simulink model "Speed_Controller_Test"  (Simulink 7.2)
settings: Solver=ode4  SolverMode=SingleTasking  StartTime=0.0  StopTime=252  FixedStep=0.01  RelTol=1e-3
InitFcn:
  | tempomat_para
StopFcn:
  | clear;
values from neighbouring files (symbols this model uses):
  A = 1.9    [tempomat_para.m]
  a_Fzg_max = 2    [tempomat_para.m]
  a_Fzg_min = -2    [tempomat_para.m]
  cw = 0.32    [tempomat_para.m]
  gang = [1 2 3 4]    [tempomat_para.m]
  gang_vec = [1 2 3 4]    [tempomat_para.m]
  i_anteil = 5    [tempomat_para.m]
  i_d = 3.42    [tempomat_para.m]
  i_g = [3.91 2.17 1.37 1.00]    [tempomat_para.m]
  lambda_gang = [1.3 1.25  1.17  1.05]    [tempomat_para.m]
  m_Fzg = 1400    [tempomat_para.m]
  M_mot_max = [130 149 163 170 168 166 162 158 150 139 123 80]    [tempomat_para.m]
  M_mot_min = [0 -40]    [tempomat_para.m]
  n_mot0 = 1000    [tempomat_para.m]
  n_mot_max = 1000:500:6500    [tempomat_para.m]
  n_mot_min = [1000 6500]    [tempomat_para.m]
  p_anteil = 100    [tempomat_para.m]
  r_dyn = 0.28    [tempomat_para.m]
  rho = 1.202    [tempomat_para.m]
  t_sch = 0.2    [tempomat_para.m]
  TI = [block '/TI']    [PSTI_callback.m]
  v_Fzg_ms0 = 0    [tempomat_para.m]
undefined symbols (not defined in the file or in its folder): Drossel_mat, getdatatypespecs
libraries: simulink x116, fzgbib x3
(part 2 of 10)

== system Speed_Controller_Test/Validation and  Test Evaluation/R2 Speed Control velocity restoration time after simple  acceleration/deceleration/CC active + no target & Speed Control active & step of V_Des = |1|  with time periods >= 7s ==
  InOut Bus : Inport  OutDataType=sfix(16)  OutScaling=2^0
  Active : Constant  Value=2  OutDataType=sfix(16)  OutScaling=2^0
  Active + no target : Constant  Value=2  OutDataType=sfix(16)  OutScaling=2^0
  Bus Selector : BusSelector  OutputSignals=Inputs.v_Des,Inputs.CCMode,Inputs.Selection
  CC active & no target : Subsystem  mask(Range - Gap Absolute Tolerance){GorR=Range, AbsoluteTolerance=0}
      mask prompts: GorR "Use range or gap"; AbsoluteTolerance "Absolute Tolerance"
      mask help: Check that a signal stays inside a range or outside a gap around a reference signal. Specify the range or the gap absolute to the reference signal.
      mask init:
      | if max(get_param(gcb,'GorR') == ' ') % Gap
      |     helpVariable1 = '~=';
      | else % Range
      |     helpVariable1 = '==';
      | end
      | set_param([gcb '/Relational Operator'],'Operator',helpVariable1);
      mask StyleString: popup(Range|Gap  ),edit
      mask Display:
      | port_label('output',1,'A');
      | port_label('input',1,'Sig');
      | port_label('input',2,'Ref');
      | text(0.40,0.53,'+');
      | text(0.415,0.46,'-');
      | text(0.5,0.5,num2str(AbsoluteTolerance));
      | text(0.05,0.5,helpVariable1);
  CC active & no target1 : Subsystem  mask(Range - Gap Absolute Tolerance){GorR=Range, AbsoluteTolerance=0}
      mask prompts: GorR "Use range or gap"; AbsoluteTolerance "Absolute Tolerance"
      mask help: Check that a signal stays inside a range or outside a gap around a reference signal. Specify the range or the gap absolute to the reference signal.
      mask init:
      | if max(get_param(gcb,'GorR') == ' ') % Gap
      |     helpVariable1 = '~=';
      | else % Range
      |     helpVariable1 = '==';
      | end
      | set_param([gcb '/Relational Operator'],'Operator',helpVariable1);
      mask StyleString: popup(Range|Gap  ),edit
      mask Display:
      | port_label('output',1,'A');
      | port_label('input',1,'Sig');
      | port_label('input',2,'Ref');
      | text(0.40,0.53,'+');
      | text(0.415,0.46,'-');
      | text(0.5,0.5,num2str(AbsoluteTolerance));
      | text(0.05,0.5,helpVariable1);
  PS : Subsystem  mask(Feature layer: preconditions synchronization){NoTI=3, NoTDD=0, NoTID=0, TIdel=[0  0  0], TDDdel=[]}
      mask prompts: NoTI "Time-independent features identifiable with or without a delay (TI)"; NoTDD "Triggered features identifiable with determinate delay or without a delay (TDD)"; NoTID "Triggered features identifiable with indeterminate delay (TID)"; TIdel "Time-independent features delays (in time steps). E.g. [0 1 0] for 3 features"; TDDdel "Triggered features delays (in time steps). E.g. [0 0] for 2 features"
      mask help: Use this block for synchronizing the precondition features. For changing the block inputs, use the parameters below. The output must be used for assertions activation.
      mask init:
      | PS_init(gcb);
      mask StyleString: popup(0|1|2|3|4|5|6|7|8|9),popup(0|1|2|3|4|5|6|7|8|9),popup(0|1|2|3|4|5|6|7|8|9),edit,edit
      mask CallbackString:
      | PSTI_callback(gcb);|PSTDD_callback(gcb);|PSTID_callback(gcb);|NoTI = str2double(get_param(gcb,'NoTI'));
      | TIdel = str2num(get_param(gcb,'TIdel'));
      | if NoTI ~= length(TIdel) && NoTI ~= 0
      |     error(['The number of delays entered (' num2str(length(TIdel)) ') does not correspond to the above specified number of time-independent features (' num2str(NoTI) ').']);
      | end|NoTDD = str2double(get_param(gcb,'NoTDD'));
      | TDDdel = str2num(get_param(gcb,'TDDdel'));
      | if NoTDD ~= length(TDDdel) && NoTDD ~= 0
      |     error(['The number of delays entered (' num2str(length(TDDdel)) ') does not correspond to the above specified number of triggered features with constant delay (' num2str(NoTDD) ').']);
      | end
  Scope1 : Scope  NumInputPorts=3
      settings: TimeRange=120  YMin=-0.003370786516853574~-5~-5  YMax=0.3966292134831465~5~5  SaveName=ScopeData5  MaxDataPoints=5000000
  Speed Control active : Subsystem  mask(Range - Gap Absolute Tolerance){GorR=Range, AbsoluteTolerance=0}
      mask prompts: GorR "Use range or gap"; AbsoluteTolerance "Absolute Tolerance"
      mask help: Check that a signal stays inside a range or outside a gap around a reference signal. Specify the range or the gap absolute to the reference signal.
      mask init:
      | if max(get_param(gcb,'GorR') == ' ') % Gap
      |     helpVariable1 = '~=';
      | else % Range
      |     helpVariable1 = '==';
      | end
      | set_param([gcb '/Relational Operator'],'Operator',helpVariable1);
      mask StyleString: popup(Range|Gap  ),edit
      mask Display:
      | port_label('output',1,'A');
      | port_label('input',1,'Sig');
      | port_label('input',2,'Ref');
      | text(0.40,0.53,'+');
      | text(0.415,0.46,'-');
      | text(0.5,0.5,num2str(AbsoluteTolerance));
      | text(0.05,0.5,helpVariable1);
  Step with step size=|1|  and time periods >= 6s detection : Subsystem  mask(Complete step detection){Param=0}
      mask prompts: Param "Mask Parameter 1:"
  true : Constant  OutDataType=sfix(16)  OutScaling=2^0
  Activate : Outport  OutDataType=sfix(16)  OutScaling=2^0
  wires:
  PS/1(Precond) -> Activate/1
  InOut Bus/1 -> Bus Selector/1
  Bus Selector/1 -> Step with step size=|1|  and time periods >= 6s detection/1(Step)  "<v_Des>"
  Bus Selector/2 -> CC active & no target/1(Signal)  "<CCMode>"
  Active + no target/1 -> CC active & no target/2(Reference)
  Active/1 -> Speed Control active/2(Reference)
  Bus Selector/3 -> Speed Control active/1(Signal)  "<Selection>"
  Step with step size=|1|  and time periods >= 6s detection/1(Complete step) -> CC active & no target1/1(Signal)
  true/1 -> CC active & no target1/2(Reference)
  CC active & no target1/1(Activate) -> PS/1(A TI1)
  CC active & no target/1(Activate) -> PS/2(A TI2)
  Speed Control active/1(Activate) -> PS/3(A TI3)

== system Speed_Controller_Test/Validation and  Test Evaluation/R2 Speed Control velocity restoration time after simple  acceleration/deceleration/after (6 seconds)  |V_Des-V_Vhcl <= 1.4| ==
  Precond : Inport  OutDataType=sfix(16)  OutScaling=2^0
  InOut Bus : Inport  Port=2  OutDataType=sfix(16)  OutScaling=2^0
  " " : Subsystem  mask(Bound){cm=<=, Lower=1, Upper=0, Ass=[1 2], Pre=[1 2], Req=[1 2]}
      mask prompts: cm "Comparison method:"; Upper "Mask Parameter 3:"; Req "Mask Parameter 6:"
      mask help:
      | Compare a signal with a reference using the specified comparison method.
      |
      | Output verdict V and lower (LL) and upper (UL) limits for reporting.
      |
      | For '==' or '~=' use "Range - Gap"
      mask init: same as Speed_Controller_Test/Validation and  Test Evaluation/R1 Speed Control step response/Maximum overshoot < 5 &  Steady state error < 5/Maximum overshoot < 5
      mask StyleString: popup(>|>=|<=|<),edit,edit,edit,edit,edit
      mask Display:
      | port_label('output', 1, ['V']);
      | port_label('input', 1, 'Sig');
      | port_label('input', 2, 'Ref');
      | text(0.05,0.5,get_param(get_param([get_param(gcb,'Parent') '/' get_param(gcb,'Name') '/Relational Operator'],'handle'),'Operator'));
  Bus Creator : BusCreator  Inputs=1
  Bus Selector : BusSelector  OutputSignals=Inputs.v_Des,Outputs.v_Vhcl
  Bus Selector{1..4} (4 alike) : BusSelector  OutputSignals=Local verdict
  PAS1 : Subsystem  mask{AFT=TI, AFD=600}
      mask prompts: AFT "Assertion feature type:"; AFD "Assertion feature delay (in time steps)"
      mask init:
      | PAS_init(gcb);
      mask StyleString: popup(TI|TDD|TID),edit
      mask CallbackString: PAS_callback(gcb);|
  PAS2 : Subsystem  mask{AFT=TI, AFD=600}
      mask prompts: AFT "Assertion feature type:"; AFD "Assertion feature delay (in time steps)"
      mask init:
      | PAS_init(gcb);
      mask StyleString: popup(TI|TDD|TID),edit
      mask CallbackString: PAS_callback(gcb);|
  R = 2 : Subsystem
  Scope : Scope  NumInputPorts=5
      settings: YMin=-5~-5~-5~80~0  YMax=5~5~5~107.5~110  SaveName=ScopeData2  MaxDataPoints=5000000
  t1 : Constant  Value=1.4  OutDataType=sfix(16)  OutScaling=2^0
  t2 : Constant  OutDataType=sfix(16)  OutScaling=2^0
  within(20 sec)1 : Subsystem  mask(Bound){cm=<=, Lower=1, Upper=0, Ass=[1 2], Pre=[1 2], Req=[1 2]}
      mask prompts: cm "Comparison method:"; Upper "Mask Parameter 3:"; Req "Mask Parameter 6:"
      mask help:
      | Compare a signal with a reference using the specified comparison method.
      |
      | Output verdict V and lower (LL) and upper (UL) limits for reporting.
      |
      | For '==' or '~=' use "Range - Gap"
      mask init: same as Speed_Controller_Test/Validation and  Test Evaluation/R1 Speed Control step response/Maximum overshoot < 5 &  Steady state error < 5/Maximum overshoot < 5
      mask StyleString: popup(>|>=|<=|<),edit,edit,edit,edit,edit
      mask Display:
      | port_label('output', 1, ['V']);
      | port_label('input', 1, 'Sig');
      | port_label('input', 2, 'Ref');
      | text(0.05,0.5,get_param(get_param([get_param(gcb,'Parent') '/' get_param(gcb,'Name') '/Relational Operator'],'handle'),'Operator'));
  |V_Des-V_Vhcl| : Subsystem
  VF info : Outport  OutDataType=sfix(16)  OutScaling=2^0
  wires:
  t1/1 -> " "/2(Reference)
  " "/1(V) -> Bus Selector1/1, PAS1/2(V)
  InOut Bus/1 -> |V_Des-V_Vhcl|/1(InOut Bus), Bus Selector/1, R = 2/2(In2)
  Bus Creator/1 -> VF info/1
  Precond/1 -> PAS1/1(Precond), PAS2/1(Precond), R = 2/1(In1)
  PAS1/1(VF Info) -> Bus Creator/1, Bus Selector2/1
  |V_Des-V_Vhcl|/1(Out1) -> " "/1(Signal)
  t2/1 -> within(20 sec)1/2(Reference)
  within(20 sec)1/1(V) -> Bus Selector4/1, PAS2/2(V)
  R = 2/1(Out1) -> within(20 sec)1/1(Signal), Scope/3
  Bus Selector4/1 -> Scope/1  "<Local verdict>"
  PAS2/1(VF Info) -> Bus Selector3/1
  Bus Selector3/1 -> Scope/2  "<Local verdict>"

== system Speed_Controller_Test/Speed control/Compute SUC inputs/neg_Beschleunigungsbegrenzung/Reset M_Br2 ==
  M_Br_n : Inport  OutDataType=sfix(16)  OutScaling=2^0
  a_Fzg_mss : Inport  Port=2  OutDataType=sfix(16)  OutScaling=2^0
  Enable : EnablePort
  Constant1 : Constant  Value=a_Fzg_min  OutDataType=sfix(16)  OutScaling=2^0
  Constant2 : Constant  Value=10  OutDataType=sfix(16)  OutScaling=2^0
  Data Store Write : DataStoreWrite  DataStoreName=M_Br2  SampleTime=-1
  Product : Product  OutDataType=sfix(16)  OutScaling=2^0  SaturateOnIntegerOverflow=on  InputSameDT=on  OutDataTypeStr=Inherit: Same as first input
  Sum : Sum  OutDataType=sfix(16)  OutScaling=2^0  SaturateOnIntegerOverflow=on  InputSameDT=on  OutDataTypeStr=Inherit: Same as first input
  Sum1 : Sum  Inputs=+-  OutDataType=sfix(16)  OutScaling=2^0  SaturateOnIntegerOverflow=on  InputSameDT=on  OutDataTypeStr=Inherit: Same as first input
  wires:
  Sum/1 -> Data Store Write/1
  M_Br_n/1 -> Sum/1
  Sum1/1 -> Product/2
  a_Fzg_mss/1 -> Sum1/1
  Constant1/1 -> Sum1/2
  Constant2/1 -> Product/1
  Product/1 -> Sum/2

== system Speed_Controller_Test/Speed control/Compute SUC inputs/pos_Beschleunigungsbegrenzung/Reset M_Mot2 ==
  M_Mot_n : Inport  OutDataType=sfix(16)  OutScaling=2^0
  Enable : EnablePort
  Data Store Write : DataStoreWrite  DataStoreName=M_Mot2  SampleTime=-1
  wires:
  M_Mot_n/1 -> Data Store Write/1

== system Speed_Controller_Test/Speed control/Speed controller/Stoergroessenkompensation/Luft- und Rollwiderstand ==
  note: Keine Steigung beruecksichtigt
  v_Fzg : Inport  OutDataType=sfix(16)  OutScaling=2^0
  F_L Berechnung : Fcn  Expr=u*rho*A/2*cw
  F_R Berechnung : Fcn  Expr=(u>0.1)*f_r*m_Fzg*g
  Fcn : Fcn  Expr=u*r_dyn
  Product : Product  OutDataType=sfix(16)  OutScaling=2^0  SaturateOnIntegerOverflow=on  InputSameDT=on  OutDataTypeStr=Inherit: Same as first input
  Sum : Sum  OutDataType=sfix(16)  OutScaling=2^0  SaturateOnIntegerOverflow=on  InputSameDT=on  OutDataTypeStr=Inherit: Same as first input
  M_G : Outport  OutDataType=sfix(16)  OutScaling=2^0  InitialOutput=0
  wires:
  Product/1 -> F_L Berechnung/1
  v_Fzg/1 -> Product/2, Product/1, F_R Berechnung/1
  F_R Berechnung/1 -> Sum/2
  F_L Berechnung/1 -> Sum/1
  Sum/1 -> Fcn/1
  Fcn/1 -> M_G/1

== system Speed_Controller_Test/Speed control/Speed controller/Stoergroessenkompensation/Sollverhalten Fahrzeug mit P-Regler1 ==
  v_soll : Inport  OutDataType=sfix(16)  OutScaling=2^0
  v_Fzg : Inport  Port=2  OutDataType=sfix(16)  OutScaling=2^0
  GR_aktiv_l : Inport  Port=3  OutDataType=sfix(16)  OutScaling=2^0
  1/T : Fcn  Expr=1/u
  Grenze3 : Constant  Value=r_dyn*m_Fzg/p_anteil  OutDataType=sfix(16)  OutScaling=2^0
  Grenze4 : Constant  Value=0.1  OutDataType=sfix(16)  OutScaling=2^0
  Integrator : Integrator  InitialCondition=v_Fzg_ms0
  Product : Product  OutDataType=sfix(16)  OutScaling=2^0  SaturateOnIntegerOverflow=on  InputSameDT=on  OutDataTypeStr=Inherit: Same as first input
  Reglerabweichung : Sum  Inputs=-+  OutDataType=sfix(16)  OutScaling=2^0  SaturateOnIntegerOverflow=on  InputSameDT=on  OutDataTypeStr=Inherit: Same as first input
  Switch : Switch  Threshold=0.5  SaturateOnIntegerOverflow=on  InputSameDT=on
  Switch1 : Switch  Threshold=0.5  SaturateOnIntegerOverflow=on  InputSameDT=on
  v_Fzg1 : Outport  OutDataType=sfix(16)  OutScaling=2^0  InitialOutput=0
  wires:
  GR_aktiv_l/1 -> Switch1/2, Switch/2
  v_Fzg/1 -> Switch1/3
  v_soll/1 -> Switch1/1
  Switch1/1 -> Reglerabweichung/2
  Grenze3/1 -> Switch/1
  Grenze4/1 -> Switch/3
  1/T/1 -> Product/2
  Reglerabweichung/1 -> Product/1
  Switch/1 -> 1/T/1
  Product/1 -> Integrator/1
  Integrator/1 -> Reglerabweichung/1, v_Fzg1/1

== system Speed_Controller_Test/Speed control/Vehicle model/Fahrzeugmodell/Drosselklappenstellung ==
  n_mot : Inport  OutDataType=sfix(16)  OutScaling=2^0
  M_Mot_b : Inport  Port=2  OutDataType=sfix(16)  OutScaling=2^0
  schalt_l : Inport  Port=3  OutDataType=sfix(16)  OutScaling=2^0
  Constant : Constant  Value=0  OutDataType=sfix(16)  OutScaling=2^0
  Constant1 : Constant  Value=n_mot0+100  OutDataType=sfix(16)  OutScaling=2^0
  Constant2 : Constant  Value=0  OutDataType=sfix(16)  OutScaling=2^0
  Drosselklappenkennfeld : Lookup2D  RowIndex=n_Mot_vec  ColumnIndex=M_Mot_vec  Table=Drossel_mat  OutDataType=sfix(16)  OutScaling=2^0  SaturateOnIntegerOverflow=on  InputSameDT=on
  Logical Operator : Logic
  Logical Operator1 : Logic  Operator=OR
  PT1 Filterung : TransferFcn  Denominator=[0.1 1]
  Relational Operator : RelationalOperator  InputSameDT=on
  Relational Operator1 : RelationalOperator  Operator=<=  InputSameDT=on
  Saturation : Saturate  UpperLimit=90  LowerLimit=0
  Switch : Switch  Threshold=0.5  SaturateOnIntegerOverflow=on  InputSameDT=on
  damit bei Vollast 90 Grad : Fcn  Expr=u+3
  DK_Stellung [Grad] : Outport  OutDataType=sfix(16)  OutScaling=2^0  InitialOutput=0
  wires:
  Relational Operator1/1 -> Logical Operator/2
  Relational Operator/1 -> Logical Operator/1
  Logical Operator/1 -> Logical Operator1/1
  schalt_l/1 -> Logical Operator1/2
  Constant/1 -> Switch/1
  Logical Operator1/1 -> Switch/2
  Constant2/1 -> Relational Operator1/2
  Constant1/1 -> Relational Operator/2
  Saturation/1 -> PT1 Filterung/1
  PT1 Filterung/1 -> DK_Stellung [Grad]/1
  Switch/1 -> Saturation/1
  M_Mot_b/1 -> Relational Operator1/1, Drosselklappenkennfeld/2
  n_mot/1 -> Relational Operator/1, Drosselklappenkennfeld/1
  Drosselklappenkennfeld/1 -> damit bei Vollast 90 Grad/1
  damit bei Vollast 90 Grad/1 -> Switch/3

== system Speed_Controller_Test/Speed control/Vehicle model/Fahrzeugmodell/Fahrwiderstaende ==
  note: Widerstandskraefte
  note: Keine Steigung beruecksichtigt
  M_Mot_b : Inport  OutDataType=sfix(16)  OutScaling=2^0
  M_Br_b : Inport  Port=2  OutDataType=sfix(16)  OutScaling=2^0
  Gang_w : Inport  Port=3  OutDataType=sfix(16)  OutScaling=2^0
  v_Fzg_ms : Inport  Port=4  OutDataType=sfix(16)  OutScaling=2^0
  F_A Berechnung ausgekuppelt : Constant  Value=0  OutDataType=sfix(16)  OutScaling=2^0
  F_A Berechnung eingekuppelt : Fcn  Expr=u[1]*u[2]*i_d/r_dyn
  F_Brems Berechnung : Fcn  Expr=(u[1]>0)*u[2]/r_dyn
  F_L Berechnung : Fcn  Expr=u*rho*A/2*cw
  F_R Berechnung : Fcn  Expr=(u>0.1)*f_r*m_Fzg*g
  Gesamtgetriebe- uebersetzung : Fcn  Expr=u*i_d
  Getriebeuebersetzung : Lookup  InputValues=gang  Table=i_g  OutDataType=sfix(16)  OutScaling=2^0  SaturateOnIntegerOverflow=on
  Mux : Mux  Inputs=2
  Mux1 : Mux  Inputs=2
  Product : Product  OutDataType=sfix(16)  OutScaling=2^0  SaturateOnIntegerOverflow=on  InputSameDT=on  OutDataTypeStr=Inherit: Same as first input
  Schaltdauer : Subsystem
  Switch : Switch  Threshold=0.5  SaturateOnIntegerOverflow=on  InputSameDT=on
  Zeit bis Gang  eingelegt ist : TransportDelay  DelayTime=t_sch  InitialOutput=1
  tw3 : ToWorkspace  VariableName=k_l  SaveFormat=Array
      settings: MaxDataPoints=speicher
  F_A : Outport  OutDataType=sfix(16)  OutScaling=2^0  InitialOutput=0
  F_L : Outport  Port=2  OutDataType=sfix(16)  OutScaling=2^0  InitialOutput=0
  F_R : Outport  Port=3  OutDataType=sfix(16)  OutScaling=2^0  InitialOutput=0
  F_Brems : Outport  Port=4  OutDataType=sfix(16)  OutScaling=2^0  InitialOutput=0
  i_gesamt : Outport  Port=5  OutDataType=sfix(16)  OutScaling=2^0  InitialOutput=0
  Gang_i : Outport  Port=6  OutDataType=sfix(16)  OutScaling=2^0  InitialOutput=0
  schalt_l : Outport  Port=7  OutDataType=sfix(16)  OutScaling=2^0  InitialOutput=0
  wires:
  F_L Berechnung/1 -> F_L/1
  Product/1 -> F_L Berechnung/1
  v_Fzg_ms/1 -> Product/2, Product/1, F_R Berechnung/1, Mux1/1
  F_Brems Berechnung/1 -> F_Brems/1
  F_R Berechnung/1 -> F_R/1
  Mux1/1 -> F_Brems Berechnung/1
  M_Br_b/1 -> Mux1/2
  Schaltdauer/1(k_l) -> schalt_l/1, Switch/2, tw3/1
  F_A Berechnung eingekuppelt/1 -> Switch/3
  M_Mot_b/1 -> Mux/2
  Mux/1 -> F_A Berechnung eingekuppelt/1
  Gesamtgetriebe- uebersetzung/1 -> i_gesamt/1
  Getriebeuebersetzung/1 -> Mux/1, Gesamtgetriebe- uebersetzung/1
  Switch/1 -> F_A/1
  Gang_w/1 -> Getriebeuebersetzung/1, Schaltdauer/1(Gang_w), Zeit bis Gang  eingelegt ist/1
  F_A Berechnung ausgekuppelt/1 -> Switch/1
  Zeit bis Gang  eingelegt ist/1 -> Gang_i/1

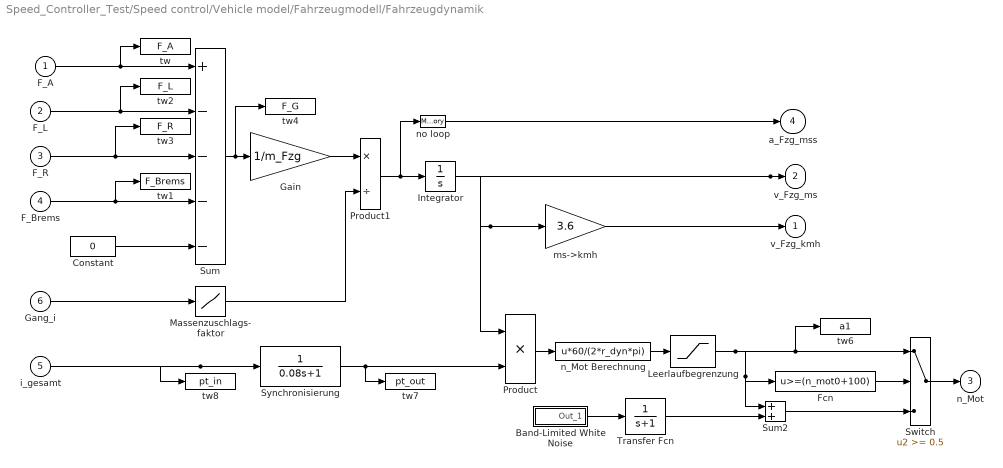
== system Speed_Controller_Test/Speed control/Vehicle model/Fahrzeugmodell/Fahrzeugdynamik ==
  F_A : Inport  OutDataType=sfix(16)  OutScaling=2^0
  F_L : Inport  Port=2  OutDataType=sfix(16)  OutScaling=2^0
  F_R : Inport  Port=3  OutDataType=sfix(16)  OutScaling=2^0
  F_Brems : Inport  Port=4  OutDataType=sfix(16)  OutScaling=2^0
  i_gesamt : Inport  Port=5  OutDataType=sfix(16)  OutScaling=2^0
  Gang_i : Inport  Port=6  OutDataType=sfix(16)  OutScaling=2^0
  Band-Limited White Noise : Subsystem  mask(Continuous White Noise.){@1=[3], @2=0.2, @3=[23341]}
      mask prompts: @1 "Noise Power:"; @2 "Sample Time:"; @3 "Seed"
      mask help:
      | White noise for continuous (s-domain) systems.
      | Band-limited using zero-order-hold.
      mask init:
      | Cov = @1; Ts = @2; seed = @3; r = rand(1,12); r2 = [r(1),r;r,r(12)]; t =[1:13;1:13];
      mask Help: Implemented using white noise into Zero-Order Hold block. The seed and power can be vectors of the same length to produce a vector of white noise sources. For faster simulation, set sample time to the highest value possible but in accordance with the fastest dynamics of system.
      mask Display: plot(t(:),r2(:))
  Constant : Constant  Value=0  OutDataType=sfix(16)  OutScaling=2^0
  Fcn : Fcn  Expr=u>=(n_mot0+100)
  Gain : Gain  Gain=1/m_Fzg  ParameterDataType=sfix(16)  ParameterScaling=2^0  OutDataType=sfix(16)  OutScaling=2^0  SaturateOnIntegerOverflow=on  OutDataTypeStr=Inherit: Same as input  ParamDataTypeStr=Inherit: Same as input
  Integrator : Integrator  InitialCondition=v_Fzg_ms0  UpperSaturationLimit=100  LowerSaturationLimit=0
  Leerlaufbegrenzung : Saturate  UpperLimit=7000  LowerLimit=n_mot0
  Massenzuschlags- faktor : Lookup  InputValues=gang_vec  Table=lambda_gang  OutDataType=sfix(16)  OutScaling=2^0  SaturateOnIntegerOverflow=on
  Product : Product  OutDataType=sfix(16)  OutScaling=2^0  SaturateOnIntegerOverflow=on  InputSameDT=on  OutDataTypeStr=Inherit: Same as first input
  Product1 : Product  Inputs=*/  OutDataType=sfix(16)  OutScaling=2^0  SaturateOnIntegerOverflow=on  InputSameDT=on  OutDataTypeStr=Inherit: Same as first input
  Sum : Sum  Inputs=+----  OutDataType=sfix(16)  OutScaling=2^0  SaturateOnIntegerOverflow=on  InputSameDT=on  OutDataTypeStr=Inherit: Same as first input
  Sum2 : Sum  OutDataType=sfix(16)  OutScaling=2^0  SaturateOnIntegerOverflow=on  InputSameDT=on  OutDataTypeStr=Inherit: Same as first input
  Switch : Switch  Threshold=0.5  SaturateOnIntegerOverflow=on  InputSameDT=on
  Synchronisierung : TransferFcn  Denominator=[0.08 1]
  Transfer Fcn : TransferFcn  Denominator=[1 1]
  ms->kmh : Gain  Gain=3.6  ParameterDataType=sfix(16)  ParameterScaling=2^0  OutDataType=sfix(16)  OutScaling=2^0  SaturateOnIntegerOverflow=on  OutDataTypeStr=Inherit: Same as input  ParamDataTypeStr=Inherit: Same as input
  n_Mot Berechnung : Fcn  Expr=u*60/(2*r_dyn*pi)
  no loop : Memory
  tw : ToWorkspace  VariableName=F_A  SaveFormat=Array
      settings: MaxDataPoints=speicher
  tw1 : ToWorkspace  VariableName=F_Brems  SaveFormat=Array
      settings: MaxDataPoints=speicher
  tw2 : ToWorkspace  VariableName=F_L  SaveFormat=Array
      settings: MaxDataPoints=speicher
  tw3 : ToWorkspace  VariableName=F_R  SaveFormat=Array
      settings: MaxDataPoints=speicher
  tw4 : ToWorkspace  VariableName=F_G  SaveFormat=Array
      settings: MaxDataPoints=speicher
  tw6 : ToWorkspace  VariableName=a1  SaveFormat=Array
      settings: MaxDataPoints=speicher
  tw7 : ToWorkspace  VariableName=pt_out  SaveFormat=Array
      settings: MaxDataPoints=speicher
  tw8 : ToWorkspace  VariableName=pt_in  SaveFormat=Array
      settings: MaxDataPoints=speicher
  v_Fzg_kmh : Outport  OutDataType=sfix(16)  OutScaling=2^0  InitialOutput=0
  v_Fzg_ms : Outport  Port=2  OutDataType=sfix(16)  OutScaling=2^0  InitialOutput=0
  n_Mot : Outport  Port=3  OutDataType=sfix(16)  OutScaling=2^0  InitialOutput=0
  a_Fzg_mss : Outport  Port=4  OutDataType=sfix(16)  OutScaling=2^0  InitialOutput=0
  wires:
  Constant/1 -> Sum/5
  F_Brems/1 -> tw1/1, Sum/4
  F_R/1 -> Sum/3, tw3/1
  F_L/1 -> Sum/2, tw2/1
  F_A/1 -> tw/1, Sum/1
  ms->kmh/1 -> v_Fzg_kmh/1
  Integrator/1 -> Product/1, ms->kmh/1, v_Fzg_ms/1
  no loop/1 -> a_Fzg_mss/1
  Product/1 -> n_Mot Berechnung/1
  n_Mot Berechnung/1 -> Leerlaufbegrenzung/1
  Gang_i/1 -> Massenzuschlags- faktor/1
  Massenzuschlags- faktor/1 -> Product1/2
  Product1/1 -> no loop/1, Integrator/1
  Gain/1 -> Product1/1
  Sum/1 -> Gain/1, tw4/1
  Synchronisierung/1 -> Product/2, tw7/1
  i_gesamt/1 -> Synchronisierung/1, tw8/1
  Fcn/1 -> Switch/2
  Sum2/1 -> Switch/3
  Leerlaufbegrenzung/1 -> tw6/1, Switch/1, Sum2/1, Fcn/1
  Transfer Fcn/1 -> Sum2/2
  Band-Limited White Noise/1(Out_1) -> Transfer Fcn/1
  Switch/1 -> n_Mot/1

== system Speed_Controller_Test/TestData 1/R1 Speed Control step response/Complete step & CC active + no target & Speed Control active/Generate complete step ==
  Out Bus : Inport  OutDataType=sfix(16)  OutScaling=2^0
  " " : RelationalOperator  Operator===  LogicOutDataTypeMode=boolean  OutDataTypeStr=boolean
  Bus Selector : BusSelector  OutputSignals=signal2.signal1.signal1.signal2.T
  Clock1 : Clock
      settings: Decimation=10
  Data Store : DataStoreMemory  DataStoreName=triggerTime  OutDataType=sfix(16)  OutScaling=2^0
  Generate step : Step  InitFcn=triggerTime=150  Time=85.4+const  Before=XF  After=XF+size  SampleTime=0  VectorParams1D=off
  "Generate step " : Step  Time=t  Before=XO  After=XF  SampleTime=0
  Hold Time : Subsystem  TreatAsAtomicUnit=on
  Hold Value : Subsystem  TreatAsAtomicUnit=on
  Memory : Memory
  Switch : Switch  Criteria=u2 > Threshold
  triggered : Constant  OutDataType=sfix(16)  OutScaling=2^0
  v_Des : Outport  OutDataType=sfix(16)  OutScaling=2^0
  wires:
  Out Bus/1 -> Bus Selector/1
  triggered/1 -> " "/2
  " "/1 -> Hold Value/1(trigger), Hold Value/Enable, Hold Time/Enable
  Generate step/1 -> Switch/1
  "Generate step "/1 -> Switch/3
  Switch/1 -> v_Des/1
  Hold Value/1(triggered) -> Switch/2
  Clock1/1 -> Hold Time/1(Clock)
  Memory/1 -> " "/1
  Bus Selector/1 -> Memory/1  "<T>"

== system Speed_Controller_Test/TestData 1/R2 Speed Control velocity restoration/ CC active + no target & Speed Control active/V_Des increases/decreases  7 times by 1 unit ==
  Generate step : Step  InitFcn=triggerTime=150  Time=147+7  Before=50  After=51  SampleTime=0  VectorParams1D=off
  Generate step1 : Step  InitFcn=triggerTime=150  Time=147+7+42+7  After=-1  SampleTime=0  VectorParams1D=off
  Step : Step  Time=147+7+21  SampleTime=0
  Step1 : Step  Time=147+7+35  SampleTime=0
  Step10 : Step  Time=147+7+42+7+28  After=-1  SampleTime=0
  Step11 : Step  Time=147+7+42+7+42  After=-1  SampleTime=0
  Step2 : Step  Time=147+7+14  SampleTime=0
  Step3 : Step  Time=147+7+7  SampleTime=0
  Step4 : Step  Time=147+7+42+7+21  After=-1  SampleTime=0
  Step5 : Step  Time=147+7+28  SampleTime=0
  Step6 : Step  Time=147+7+42  SampleTime=0
  Step7 : Step  Time=147+7+42+7+35  After=-1  SampleTime=0
  Step8 : Step  Time=147+7+42+7+14  After=-2  SampleTime=0
  Step9 : Step  Time=147+7+42+7+7  After=-1  SampleTime=0
  Sum1 : Sum  Inputs=+++++++  OutDataType=sfix(16)  OutScaling=2^0
  Sum2 : Sum  Inputs=+++++++  OutDataType=sfix(16)  OutScaling=2^0
  Sum3 : Sum  OutDataType=sfix(16)  OutScaling=2^0
  v_Des : Outport  OutDataType=sfix(16)  OutScaling=2^0
  wires:
  Sum2/1 -> Sum3/1
  Sum1/1 -> Sum3/2
  Sum3/1 -> v_Des/1
  Generate step/1 -> Sum1/1
  Step3/1 -> Sum1/2
  Step2/1 -> Sum1/3
  Step/1 -> Sum1/4
  Step5/1 -> Sum1/5
  Step1/1 -> Sum1/6
  Step6/1 -> Sum1/7
  Generate step1/1 -> Sum2/1
  Step9/1 -> Sum2/2
  Step8/1 -> Sum2/3
  Step4/1 -> Sum2/4
  Step10/1 -> Sum2/5
  Step7/1 -> Sum2/6
  Step11/1 -> Sum2/7

== system Speed_Controller_Test/Validation and  Test Evaluation/R1 Speed Control step response/Complete step & CC active + no target & Speed Control active/CC active & no target ==
  Signal : Inport  OutDataType=sfix(16)  OutScaling=2^0
  Reference : Inport  Port=2  OutDataType=sfix(16)  OutScaling=2^0
  Abs : Abs
  Abs1 : Abs
  Absolute Tolerance : Constant  Value=AbsoluteTolerance  OutDataType=sfix(16)  OutScaling=2^0
  Add : Sum  Inputs=+-  OutDataType=sfix(16)  OutScaling=2^-10
  Relational Operator : RelationalOperator  Operator===  LogicOutDataTypeMode=boolean  OutDataTypeStr=boolean
  Activate : Outport  OutDataType=sfix(16)  OutScaling=2^0
  wires:
  Relational Operator/1 -> Activate/1
  Abs/1 -> Relational Operator/1
  Add/1 -> Abs/1
  Signal/1 -> Add/1
  Reference/1 -> Add/2
  Absolute Tolerance/1 -> Abs1/1
  Abs1/1 -> Relational Operator/2

== system Speed_Controller_Test/Validation and  Test Evaluation/R1 Speed Control step response/Complete step & CC active + no target & Speed Control active/Complete step detection ==
  Step : Inport  OutDataType=sfix(16)  OutScaling=2^0
  Step response : Inport  Port=2  OutDataType=sfix(16)  OutScaling=2^0
  Step detection : Subsystem  mask{MT=10, RT=0.001}
      mask prompts: MT "Minimal time for signals to be constant before a step"; RT "Relative tolerance for constant detection in %"
      mask CallbackString:
      | if (str2double(get_param(gcb,'MT')) < 0)
      |     error(['Minimal time specified (' get_param(gcb,'MT') ') negative. Please give a non-negative value.']);
      | else
      |     set_param([gcb '/Active if signals constant for some specified time/Min Time'],'Value',get_param(gcb,'MT'));
      | end|if or( (str2double(get_param(gcb,'RT')) < 0), (str2double(get_param(gcb,'RT')) > 100))
      |     error(['Relative tolerance value (' get_param(gcb,'RT') ') out of range. Please give a value between 0 and 100.']);
      | else
      |     set_param([gcb '/Active if signals constant for some specified time/Time since signal constant/Detect constant/Relative tolerance/Relative Tolerance'],'Value',get_param(gcb,'RT'));
      |     set_param([gcb '/Active if signals constant for some specified time/Time since signal constant/Detect constant'],'RT',get_param(gcb,'RT'));
      |     set_param([gcb '/Active if signals constant for some specified time/Time since signal constant'],'RT',get_param(gcb,'RT'));
      |     set_param([gcb '/Active if signals constant for some specified time/Time since signal constant1/Detect constant/Relative tolerance/Relative Tolerance'],'Value',get_param(gcb,'RT'));
      |     set_param([gcb '/Active if signals constant for some specified time/Time since signal constant1/Detect constant'],'RT',get_param(gcb,'RT'));
      |     set_param([gcb '/Active if signals constant for some specified time/Time since signal constant1'],'RT',get_param(gcb,'RT'));
      | end
  Step detection reset : Subsystem  mask{MT=10, RT=0.0001, MSS=10}
      mask prompts: MT "Minimal time for signals to be constant before a step"; RT "Relative tolerance for constant detection in %"; MSS "Minimal step size for step detection"
      mask CallbackString:
      | if (str2double(get_param(gcb,'MT')) < 0)
      |     error(['Minimal time specified (' get_param(gcb,'MT') ') negative. Please give a non-negative value.']);
      | else
      |     set_param([gcb '/Active if signals constant for some specified time/Min Time'],'Value',get_param(gcb,'MT'));
      | end|if or( (str2double(get_param(gcb,'RT')) < 0), (str2double(get_param(gcb,'RT')) > 100))
      |     error(['Relative tolerance value (' get_param(gcb,'RT') ') out of range. Please give a value between 0 and 100.']);
      | else
      |     set_param([gcb '/Active if signals constant for some specified time/Time since signal constant/Detect constant/Relative tolerance/Relative Tolerance'],'Value',get_param(gcb,'RT'));
      |     set_param([gcb '/Active if signals constant for some specified time/Time since signal constant/Detect constant'],'RT',get_param(gcb,'RT'));
      |     set_param([gcb '/Active if signals constant for some specified time/Time since signal constant'],'RT',get_param(gcb,'RT'));
      |     set_param([gcb '/Active if signals constant for some specified time/Time since signal constant1/Detect constant/Relative tolerance/Relative Tolerance'],'Value',get_param(gcb,'RT'));
      |     set_param([gcb '/Active if signals constant for some specified time/Time since signal constant1/Detect constant'],'RT',get_param(gcb,'RT'));
      |     set_param([gcb '/Active if signals constant for some specified time/Time since signal constant1'],'RT',get_param(gcb,'RT'));
      | end|if (str2double(get_param(gcb,'MSS')) < 0)
      |     error(['Minimal step size specified (' get_param(gcb,'MSS') ') negative. Please give a non-negative value.']);
      | else
      |     set_param([gcb '/Step detection/Min step size'],'Value',get_param(gcb,'MSS'));
      |     set_param([gcb '/Step detection'],'StepSize',get_param(gcb,'MSS'));
      | 
      | end
  R : Outport  OutDataType=sfix(16)  OutScaling=2^0
  T : Outport  Port=2  OutDataType=sfix(16)  OutScaling=2^0
  Complete step : Outport  Port=3  OutDataType=sfix(16)  OutScaling=2^0
  wires:
  Step/1 -> Step detection/2(Step), Step detection reset/1(Step)
  Step response/1 -> Step detection/3(Step response), Step detection reset/2(Step response)
  Step detection reset/1(R) -> Step detection/1(R), R/1
  Step detection/1(End of complete step) -> Complete step/1, T/1

== system Speed_Controller_Test/Validation and  Test Evaluation/R1 Speed Control step response/Complete step & CC active + no target & Speed Control active/PS ==
  R TID1 : Inport  OutDataType=sfix(16)  OutScaling=2^0
  T TID1 : Inport  Port=2  OutDataType=sfix(16)  OutScaling=2^0
  A TID1 : Inport  Port=3  OutDataType=sfix(16)  OutScaling=2^0
  A TI1 : Inport  Port=4  OutDataType=sfix(16)  OutScaling=2^0
  A TI2 : Inport  Port=5  OutDataType=sfix(16)  OutScaling=2^0
  AND : Logic  Inputs=4  AllPortsSameDT=off  OutDataTypeMode=boolean  OutDataTypeStr=boolean
  Bus Creator : BusCreator  Inputs=3
  Data Type Conversion : DataTypeConversion  OutDataType=sfix(16)  OutScaling=2^0
  Data Type Conversion1 : DataTypeConversion  OutDataType=sfix(16)  OutScaling=2^0
  Data Type Conversion2 : DataTypeConversion  OutDataType=sfix(16)  OutScaling=2^0
  Max Delay A : Subsystem  TreatAsAtomicUnit=on  mask{Delay=0}
      mask prompts: Delay "Delay (in simulation steps) for the input signal:"
      mask init:
      | %set_param([gcb '/Discrete Transfer Fcn'],'Denominator',['[' num2str([1 zeros(1,str2double(get_param(gcb,'Delay')))]) ']']);
      mask CallbackString:
      | Delay = str2double(get_param(gcb,'Delay'));
      | if Delay < 0
      |     set_param(gcb,'Delay','0');
      |     error('Only non-negative delays are possible (causality).');
      |     set_param([gcb '/Delay'],'Value','0');
      | elseif Delay == 0
      |     set_param([gcb '/Delay'],'Value','0');
      | else
      |     set_param([gcb '/Integer Delay'],'NumDelays',num2str(Delay));
      |     set_param([gcb '/Delay'],'Value',num2str(Delay));
      | end
      mask Display: text(0.5,0.5,['z^{ ' num2str((-1)*str2double(get_param(gcb,'Delay'))) '}'],'texmode','on');
  Max Delay R : Subsystem  TreatAsAtomicUnit=on  mask{Delay=0}
      mask prompts: Delay "Delay (in simulation steps) for the input signal:"
      mask init:
      | %set_param([gcb '/Discrete Transfer Fcn'],'Denominator',['[' num2str([1 zeros(1,str2double(get_param(gcb,'Delay')))]) ']']);
      mask CallbackString:
      | Delay = str2double(get_param(gcb,'Delay'));
      | if Delay < 0
      |     set_param(gcb,'Delay','0');
      |     error('Only non-negative delays are possible (causality).');
      |     set_param([gcb '/Delay'],'Value','0');
      | elseif Delay == 0
      |     set_param([gcb '/Delay'],'Value','0');
      | else
      |     set_param([gcb '/Integer Delay'],'NumDelays',num2str(Delay));
      |     set_param([gcb '/Delay'],'Value',num2str(Delay));
      | end
      mask Display: text(0.5,0.5,['z^{ ' num2str((-1)*str2double(get_param(gcb,'Delay'))) '}'],'texmode','on');
  Max Delay T : Subsystem  TreatAsAtomicUnit=on  mask{Delay=0}
      mask prompts: Delay "Delay (in simulation steps) for the input signal:"
      mask init:
      | %set_param([gcb '/Discrete Transfer Fcn'],'Denominator',['[' num2str([1 zeros(1,str2double(get_param(gcb,'Delay')))]) ']']);
      mask CallbackString:
      | Delay = str2double(get_param(gcb,'Delay'));
      | if Delay < 0
      |     set_param(gcb,'Delay','0');
      |     error('Only non-negative delays are possible (causality).');
      |     set_param([gcb '/Delay'],'Value','0');
      | elseif Delay == 0
      |     set_param([gcb '/Delay'],'Value','0');
      | else
      |     set_param([gcb '/Integer Delay'],'NumDelays',num2str(Delay));
      |     set_param([gcb '/Delay'],'Value',num2str(Delay));
      | end
      mask Display: text(0.5,0.5,['z^{ ' num2str((-1)*str2double(get_param(gcb,'Delay'))) '}'],'texmode','on');
  OR - AND : Subsystem
  TDD : Subsystem
  TI : Subsystem
  TID : Subsystem
  Precond : Outport  OutDataType=sfix(16)  OutScaling=2^0
  wires:
  A TID1/1 -> TID/2(A1)
  T TID1/1 -> TID/1(T1)
  R TID1/1 -> OR - AND/1(R1)
  TDD/2(T) -> AND/4
  TID/2(T) -> Max Delay T/1(In1)
  TID/1(A) -> Max Delay A/1(In1)
  Bus Creator/1 -> Precond/1
  Data Type Conversion/1 -> Bus Creator/1  "A"
  Data Type Conversion1/1 -> Bus Creator/2  "T"
  TDD/1(A) -> AND/3
  Max Delay T/1(Out1) -> Data Type Conversion1/1
  Max Delay R/1(Out1) -> AND/1
  Max Delay A/1(Out1) -> Data Type Conversion/1
  AND/1 -> Data Type Conversion2/1
  OR - AND/2(AND) -> TID/4(R AND), Max Delay R/1(In1)
  OR - AND/1(OR) -> TID/3(R OR)
  TI/1(A) -> AND/2
  Data Type Conversion2/1 -> Bus Creator/3  "R"
  A TI1/1 -> TI/1(A1)
  A TI2/1 -> TI/2(A2)

== system Speed_Controller_Test/Validation and  Test Evaluation/R1 Speed Control step response/Complete step & CC active + no target & Speed Control active/Range - Gap Absolute tolerance Precond ==
  Signal : Inport  OutDataType=sfix(16)  OutScaling=2^0
  Reference : Inport  Port=2  OutDataType=sfix(16)  OutScaling=2^0
  Abs : Abs
  Abs1 : Abs
  Absolute Tolerance : Constant  Value=AbsoluteTolerance  OutDataType=sfix(16)  OutScaling=2^0
  Add : Sum  Inputs=+-  OutDataType=sfix(16)  OutScaling=2^-10
  Relational Operator : RelationalOperator  Operator===  LogicOutDataTypeMode=boolean  OutDataTypeStr=boolean
  Activate : Outport  OutDataType=sfix(16)  OutScaling=2^0
  wires:
  Abs1/1 -> Relational Operator/2
  Absolute Tolerance/1 -> Abs1/1
  Reference/1 -> Add/2
  Signal/1 -> Add/1
  Add/1 -> Abs/1
  Abs/1 -> Relational Operator/1
  Relational Operator/1 -> Activate/1

== system Speed_Controller_Test/Validation and  Test Evaluation/R1 Speed Control step response/Complete step & CC active + no target & Speed Control active/Speed control active ==
  Signal : Inport  OutDataType=sfix(16)  OutScaling=2^0
  Reference : Inport  Port=2  OutDataType=sfix(16)  OutScaling=2^0
  Abs : Abs
  Abs1 : Abs
  Absolute Tolerance : Constant  Value=AbsoluteTolerance  OutDataType=sfix(16)  OutScaling=2^0
  Add : Sum  Inputs=+-  OutDataType=sfix(16)  OutScaling=2^-10
  Relational Operator : RelationalOperator  Operator===  LogicOutDataTypeMode=boolean  OutDataTypeStr=boolean
  Activate : Outport  OutDataType=sfix(16)  OutScaling=2^0
  wires:
  Abs1/1 -> Relational Operator/2
  Absolute Tolerance/1 -> Abs1/1
  Reference/1 -> Add/2
  Signal/1 -> Add/1
  Add/1 -> Abs/1
  Abs/1 -> Relational Operator/1
  Relational Operator/1 -> Activate/1

== system Speed_Controller_Test/Validation and  Test Evaluation/R1 Speed Control step response/Maximum overshoot < 5 &  Steady state error < 5/Maximum overshoot < 5 ==
  Signal : Inport  OutDataType=sfix(16)  OutScaling=2^0
  Reference : Inport  Port=2  OutDataType=sfix(16)  OutScaling=2^0
  Bus Creator : BusCreator  Inputs=5
  Data Type Conversion{,1..3} (4 alike) : DataTypeConversion  OutDataType=sfix(16)  OutScaling=2^0
  Delay : Constant  Value=0  OutDataType=sfix(16)  OutScaling=2^0
  LOWER : Constant  Value=Lower  OutDataTypeMode=int8  OutDataType=sfix(16)  OutScaling=2^0  OutDataTypeStr=int8
  No Limit : Constant  Value=Inf  OutDataType=sfix(16)  OutScaling=2^0
  No limit : Constant  Value=-Inf  OutDataType=sfix(16)  OutScaling=2^0
  Relational Operator : RelationalOperator  Operator=<  LogicOutDataTypeMode=boolean  LogicDataType=double  OutDataTypeStr=boolean
  Switch 2 : Switch  Criteria=u2 ~= 0
  Switch 3 : Switch  Criteria=u2 ~= 0
  UPPER : Constant  Value=Upper  OutDataTypeMode=int8  OutDataType=sfix(16)  OutScaling=2^0  OutDataTypeStr=int8
  V : Outport  OutDataType=sfix(16)  OutScaling=2^0  InitialOutput=[2]
  wires:
  Relational Operator/1 -> Data Type Conversion/1
  Data Type Conversion3/1 -> Bus Creator/4  "Actual data"
  Data Type Conversion2/1 -> Bus Creator/3  "Expected upper limit"
  Data Type Conversion1/1 -> Bus Creator/2  "Expected lower limit"
  Data Type Conversion/1 -> Bus Creator/1  "Local verdict"
  Bus Creator/1 -> V/1
  Reference/1 -> Relational Operator/2, Switch 2/3, Switch 3/3
  Signal/1 -> Data Type Conversion3/1, Relational Operator/1
  UPPER/1 -> Switch 3/2
  No Limit/1 -> Switch 3/1
  LOWER/1 -> Switch 2/2
  No limit/1 -> Switch 2/1
  Switch 2/1 -> Data Type Conversion1/1
  Switch 3/1 -> Data Type Conversion2/1
  Delay/1 -> Bus Creator/5  "Delay"

== system Speed_Controller_Test/Validation and  Test Evaluation/R1 Speed Control step response/Maximum overshoot < 5 &  Steady state error < 5/PAS ==
  Precond : Inport  OutDataType=sfix(16)  OutScaling=2^0
  R : Inport  Port=2  OutDataType=sfix(16)  OutScaling=2^0
  T : Inport  Port=3  OutDataType=sfix(16)  OutScaling=2^0
  V : Inport  Port=4  OutDataType=sfix(16)  OutScaling=2^0
  A delay : Subsystem  TreatAsAtomicUnit=on  mask{Delay=0}
      mask prompts: Delay "Delay (in simulation steps) for the input signal:"
      mask init:
      | %set_param([gcb '/Discrete Transfer Fcn'],'Denominator',['[' num2str([1 zeros(1,str2double(get_param(gcb,'Delay')))]) ']']);
      mask CallbackString:
      | Delay = str2double(get_param(gcb,'Delay'));
      | if Delay < 0
      |     set_param(gcb,'Delay','0');
      |     error('Only non-negative delays are possible (causality).');
      |     set_param([gcb '/Delay'],'Value','0');
      | elseif Delay == 0
      |     set_param([gcb '/Delay'],'Value','0');
      | else
      |     set_param([gcb '/Integer Delay'],'NumDelays',num2str(Delay));
      |     set_param([gcb '/Delay'],'Value',num2str(Delay));
      | end
      mask Display: text(0.5,0.5,['z^{ ' num2str((-1)*str2double(get_param(gcb,'Delay'))) '}'],'texmode','on');
  AND1 : Logic  AllPortsSameDT=off  OutDataTypeMode=boolean  OutDataTypeStr=boolean
  Bus Selector : BusSelector  OutputSignals=Local verdict
  Bus Selector1 : BusSelector  OutputSignals=Expected lower limit,Expected upper limit,Actual data
  Bus Selector2 : BusSelector  OutputSignals=R,T,A
  Bus Assignment : BusAssignment  AssignedSignals=Local verdict,Delay
  Bus Assignment1 : BusAssignment  AssignedSignals=Expected lower limit,Expected upper limit,Actual data
  Constant : Constant  Value=-1  OutDataType=sfix(16)  OutScaling=2^0
  Delay bus signals : Subsystem
  Ra delay : Subsystem  TreatAsAtomicUnit=on  mask{Delay=0}
      mask prompts: Delay "Delay (in simulation steps) for the input signal:"
      mask init:
      | %set_param([gcb '/Discrete Transfer Fcn'],'Denominator',['[' num2str([1 zeros(1,str2double(get_param(gcb,'Delay')))]) ']']);
      mask CallbackString:
      | Delay = str2double(get_param(gcb,'Delay'));
      | if Delay < 0
      |     set_param(gcb,'Delay','0');
      |     error('Only non-negative delays are possible (causality).');
      |     set_param([gcb '/Delay'],'Value','0');
      | elseif Delay == 0
      |     set_param([gcb '/Delay'],'Value','0');
      | else
      |     set_param([gcb '/Integer Delay'],'NumDelays',num2str(Delay));
      |     set_param([gcb '/Delay'],'Value',num2str(Delay));
      | end
      mask Display: text(0.5,0.5,['z^{ ' num2str((-1)*str2double(get_param(gcb,'Delay'))) '}'],'texmode','on');
  Rp delay : Subsystem  TreatAsAtomicUnit=on  mask{Delay=0}
      mask prompts: Delay "Delay (in simulation steps) for the input signal:"
      mask init:
      | %set_param([gcb '/Discrete Transfer Fcn'],'Denominator',['[' num2str([1 zeros(1,str2double(get_param(gcb,'Delay')))]) ']']);
      mask CallbackString:
      | Delay = str2double(get_param(gcb,'Delay'));
      | if Delay < 0
      |     set_param(gcb,'Delay','0');
      |     error('Only non-negative delays are possible (causality).');
      |     set_param([gcb '/Delay'],'Value','0');
      | elseif Delay == 0
      |     set_param([gcb '/Delay'],'Value','0');
      | else
      |     set_param([gcb '/Integer Delay'],'NumDelays',num2str(Delay));
      |     set_param([gcb '/Delay'],'Value',num2str(Delay));
      | end
      mask Display: text(0.5,0.5,['z^{ ' num2str((-1)*str2double(get_param(gcb,'Delay'))) '}'],'texmode','on');
  Ta delay : Subsystem  TreatAsAtomicUnit=on  mask{Delay=0}
      mask prompts: Delay "Delay (in simulation steps) for the input signal:"
      mask init:
      | %set_param([gcb '/Discrete Transfer Fcn'],'Denominator',['[' num2str([1 zeros(1,str2double(get_param(gcb,'Delay')))]) ']']);
      mask CallbackString:
      | Delay = str2double(get_param(gcb,'Delay'));
      | if Delay < 0
      |     set_param(gcb,'Delay','0');
      |     error('Only non-negative delays are possible (causality).');
      |     set_param([gcb '/Delay'],'Value','0');
      | elseif Delay == 0
      |     set_param([gcb '/Delay'],'Value','0');
      | else
      |     set_param([gcb '/Integer Delay'],'NumDelays',num2str(Delay));
      |     set_param([gcb '/Delay'],'Value',num2str(Delay));
      | end
      mask Display: text(0.5,0.5,['z^{ ' num2str((-1)*str2double(get_param(gcb,'Delay'))) '}'],'texmode','on');
  Tp delay : Subsystem  TreatAsAtomicUnit=on  mask{Delay=0}
      mask prompts: Delay "Delay (in simulation steps) for the input signal:"
      mask init:
      | %set_param([gcb '/Discrete Transfer Fcn'],'Denominator',['[' num2str([1 zeros(1,str2double(get_param(gcb,'Delay')))]) ']']);
      mask CallbackString:
      | Delay = str2double(get_param(gcb,'Delay'));
      | if Delay < 0
      |     set_param(gcb,'Delay','0');
      |     error('Only non-negative delays are possible (causality).');
      |     set_param([gcb '/Delay'],'Value','0');
      | elseif Delay == 0
      |     set_param([gcb '/Delay'],'Value','0');
      | else
      |     set_param([gcb '/Integer Delay'],'NumDelays',num2str(Delay));
      |     set_param([gcb '/Delay'],'Value',num2str(Delay));
      | end
      mask Display: text(0.5,0.5,['z^{ ' num2str((-1)*str2double(get_param(gcb,'Delay'))) '}'],'texmode','on');
  V delay : Subsystem  TreatAsAtomicUnit=on  mask{Delay=0}
      mask prompts: Delay "Delay (in simulation steps) for the input signal:"
      mask init:
      | %set_param([gcb '/Discrete Transfer Fcn'],'Denominator',['[' num2str([1 zeros(1,str2double(get_param(gcb,'Delay')))]) ']']);
      mask CallbackString:
      | Delay = str2double(get_param(gcb,'Delay'));
      | if Delay < 0
      |     set_param(gcb,'Delay','0');
      |     error('Only non-negative delays are possible (causality).');
      |     set_param([gcb '/Delay'],'Value','0');
      | elseif Delay == 0
      |     set_param([gcb '/Delay'],'Value','0');
      | else
      |     set_param([gcb '/Integer Delay'],'NumDelays',num2str(Delay));
      |     set_param([gcb '/Delay'],'Value',num2str(Delay));
      | end
      mask Display: text(0.5,0.5,['z^{ ' num2str((-1)*str2double(get_param(gcb,'Delay'))) '}'],'texmode','on');
  error : Subsystem
  none - pass - fail : Subsystem
  sw D : Switch  Criteria=u2 ~= 0
  sw V : Switch  Criteria=u2 ~= 0
  VF Info : Outport  OutDataType=sfix(16)  OutScaling=2^0
  wires:
  Ta delay/1(Out1) -> none - pass - fail/5(Ta), error/5(Ta)
  Delay bus signals/3(ADout) -> Bus Assignment1/4
  Delay bus signals/2(EULout) -> Bus Assignment1/3
  Delay bus signals/1(ELLout) -> Bus Assignment1/2
  Bus Assignment1/1 -> Bus Assignment/1
  Bus Selector1/3 -> Delay bus signals/3(ADin)  "<Actual data>"
  Bus Selector1/2 -> Delay bus signals/2(EULin)  "<Expected upper limit>"
  Bus Selector1/1 -> Delay bus signals/1(ELLin)  "<Expected lower limit>"
  T/1 -> Ta delay/1(In1)
  R/1 -> Ra delay/1(In1)
  Precond/1 -> Bus Selector2/1
  AND1/1 -> none - pass - fail/7(R AND)
  Ra delay/1(Out1) -> AND1/2, none - pass - fail/4(Ra), error/4(Ra)
  V delay/1(Out1) -> none - pass - fail/6(V), error/6(V)
  A delay/1(Out1) -> none - pass - fail/3(A), error/3(A)
  Tp delay/1(Out1) -> none - pass - fail/2(Tp), error/2(Tp)
  Rp delay/1(Out1) -> AND1/1, none - pass - fail/1(Rp), error/1(Rp)
  Bus Selector2/3 -> A delay/1(In1)  "<A>"
  Bus Selector2/2 -> Tp delay/1(In1)  "<T>"
  Bus Selector2/1 -> Rp delay/1(In1)  "<R>"
  Bus Assignment/1 -> VF Info/1
  Bus Selector/1 -> V delay/1(In1)  "<Local verdict>"
  sw D/1 -> Bus Assignment/3
  sw V/1 -> Bus Assignment/2
  none - pass - fail/3(Delay) -> sw D/3
  none - pass - fail/2(MaxDelay) -> sw D/1
  none - pass - fail/1(Verdict) -> sw V/3
  Constant/1 -> sw V/1
  error/1(Verror) -> sw D/2, sw V/2
  V/1 -> Bus Assignment1/1, Bus Selector1/1, Bus Selector/1
